simulink model "PioneerROS_Controller"  (R2019b)
settings: Solver=FixedStepAuto  StartTime=0.0  StopTime=inf  FixedStep=0.1  RelTol=1e-3
libraries: robotlib x4
settings Model: SimulationMode=external  EnablePacing=on  Creator=gavin  LastModifiedBy=gavin
settings OptimizationCC: EnhancedBackFolding=on  PassReuseOutputArgsThreshold=0  MaxStackSize=64  OptimizeBlockOrder=speed  DifferentSizesBufferReuse=on  OptimizationCustomize=off
settings DebuggingCC: ParameterTunabilityLossMsg=error
settings HardwareCC: ProdBitPerPointer=32  ProdBitPerSizeT=32  ProdBitPerPtrDiffT=32  ProdLargestAtomicFloat=None  ProdIntDivRoundTo=Undefined  ProdEndianess=Unspecified  ProdWordSize=32  ProdHWDeviceType=Generic->Unspecified (assume 32-bit Generic)  UseEmbeddedCoderFeatures=off
settings SFSimCC: MATLABDynamicMemAlloc=off
settings RTWCC: SystemTargetFile=ert.tlc  HardwareBoard=Robot Operating System (ROS)  TLCOptions="-aInlineSetEventsForThisBaseRateFcn=TLC_FALSE -aSuppressMultiTaskScheduler=TLC_FALSE  -aRateBasedStepFcn=0"  TemplateMakefile=ert_default_tmf  GenerateReport=on  Toolchain=Catkin  LaunchReport=on  TargetLang=C++
settings CodeAppCC: ForceParamTrailComments=on  OperatorAnnotations=on
settings ERTTargetCC: ERTCustomFileBanners=off  SupportContinuousTime=on  SupportNonInlinedSFcns=on  RemoveResetFunc=off  ModelStepFunctionPrototypeControlCompliant=off

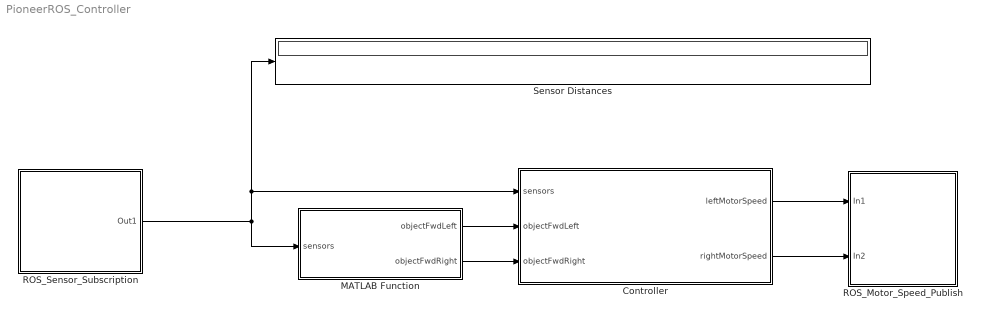
== system PioneerROS_Controller ==
  Controller : Stateflow chart  BlockKeywords=__PRM__SERIALIZED__DATA__:Stateflow Chart,Stateflow Diagram  TreatAsAtomicUnit=on
  MATLAB Function : MATLAB Function  TreatAsAtomicUnit=on
  ROS_Motor_Speed_Publish : Subsystem
  ROS_Sensor_Subscription : Subsystem
  Sensor Distances : Display
  wires:
  ROS_Sensor_Subscription/1(Out1) -> Controller/1(sensors), Sensor Distances/1, MATLAB Function/1(sensors)
  MATLAB Function/1(objectFwdLeft) -> Controller/2(objectFwdLeft)
  MATLAB Function/2(objectFwdRight) -> Controller/3(objectFwdRight)
  Controller/1(leftMotorSpeed) -> ROS_Motor_Speed_Publish/1(In1)
  Controller/2(rightMotorSpeed) -> ROS_Motor_Speed_Publish/2(In2)

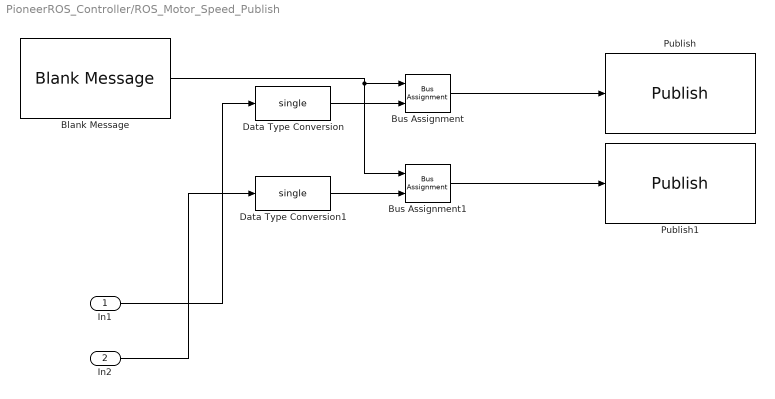
== system PioneerROS_Controller/ROS_Motor_Speed_Publish ==
  In1 : Inport
  In2 : Inport  Port=2
  Blank Message : robotlib/Blank Message  messageClass=Message  entityType=std_msgs/Float32  messageType=std_msgs/Float32  SampleTime=inf
      settings: SourceProductName=ROS Toolbox
  Bus Assignment : BusAssignment  AssignedSignals=Data
  Bus Assignment1 : BusAssignment  AssignedSignals=Data
  Data Type Conversion : DataTypeConversion  OutDataTypeStr=single
  Data Type Conversion1 : DataTypeConversion  OutDataTypeStr=single
  Publish : robotlib/Publish  topicSource=Select from ROS network  topic=/leftMotorSpeed_Bob  messageType=std_msgs/Float32  messageQueueLength=1
      settings: SourceProductName=ROS Toolbox
  Publish1 : robotlib/Publish  topicSource=Select from ROS network  topic=/rightMotorSpeed_Bob  messageType=std_msgs/Float32  messageQueueLength=1
      settings: SourceProductName=ROS Toolbox
  wires:
  In1/1 -> Data Type Conversion/1
  Bus Assignment/1 -> Publish/1
  Data Type Conversion1/1 -> Bus Assignment1/2
  Bus Assignment1/1 -> Publish1/1
  Blank Message/1 -> Bus Assignment1/1, Bus Assignment/1
  Data Type Conversion/1 -> Bus Assignment/2
  In2/1 -> Data Type Conversion1/1

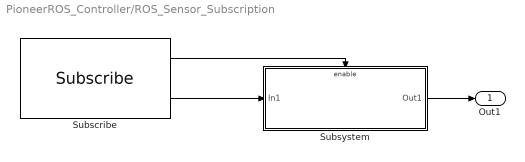
== system PioneerROS_Controller/ROS_Sensor_Subscription ==
  Subscribe : robotlib/Subscribe  topicSource=Select from ROS network  topic=/sensorTrigger_Bob  messageType=std_msgs/Float32MultiArray  sampleTime=0.1  messageQueueLength=1
      settings: SourceProductName=ROS Toolbox
  Subsystem : Subsystem
  Out1 : Outport
  wires:
  Subscribe/2 -> Subsystem/1(In1)
  Subscribe/1 -> Subsystem/Enable
  Subsystem/1(Out1) -> Out1/1

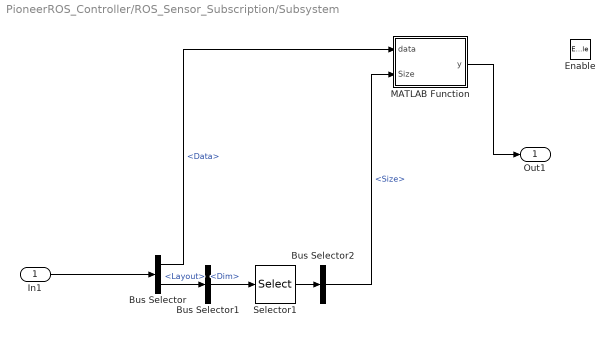
== system PioneerROS_Controller/ROS_Sensor_Subscription/Subsystem ==
  In1 : Inport
  Enable : EnablePort  PropagateVarSize=During execution
  Bus Selector : BusSelector  OutputSignals=Data,Layout
  Bus Selector1 : BusSelector  OutputSignals=Dim
  Bus Selector2 : BusSelector  OutputSignals=Size
  MATLAB Function : MATLAB Function  TreatAsAtomicUnit=on
  Selector1 : Selector  InputPortWidth=16  IndexOptions=Index vector (dialog)  Indices=[1]  OutputSizes=1
  Out1 : Outport
  wires:
  In1/1 -> Bus Selector/1
  Bus Selector1/1 -> Selector1/1  "<Dim>"
  MATLAB Function/1(y) -> Out1/1
  Bus Selector/2 -> Bus Selector1/1  "<Layout>"
  Bus Selector/1 -> MATLAB Function/1(data)  "<Data>"
  Bus Selector2/1 -> MATLAB Function/2(Size)  "<Size>"
  Selector1/1 -> Bus Selector2/1

== matlab function PioneerROS_Controller/MATLAB Function ==
  data: sensors input size=128; objectFwdLeft output size=1; objectFwdRight output size=1
function [objectFwdLeft,objectFwdRight] = fcn(sensors)
if (sensors(1) < 1) || (sensors(2) < 1) || (sensors(3) < 1) || (sensors(4) < 1)
    objectFwdLeft = 1;
else
    objectFwdLeft = 0;
end
if (sensors(5) < 1) || (sensors(6) < 1) || (sensors(7) < 1) || (sensors(8) < 1)
    objectFwdRight = 1;
else
    objectFwdRight = 0;
end

== matlab function PioneerROS_Controller/ROS_Sensor_Subscription/Subsystem/MATLAB Function ==
  data: data input; y output size=128; Size input
function y = fcn(data, Size)
%y = zeros(1,Size);
y = data(1:Size);

== stateflow chart PioneerROS_Controller/Controller ==
  state GoForwards
    en: leftMotorSpeed=1;
    en: rightMotorSpeed=1;
  state GoRight
    en: leftMotorSpeed=0.5;
    en: rightMotorSpeed=-0.5;
  state GoLeft
    en: leftMotorSpeed=-0.5;
    en: rightMotorSpeed=0.5;
  GoLeft -> GoForwards [order 3]
  (default) -> GoForwards
  GoRight -> GoForwards [order 3]
  GoForwards -> GoRight [order 2] : [objectFwdLeft]
  GoForwards -> GoLeft [order 1] : [objectFwdRight]
  GoLeft -> GoRight [order 1] : [objectFwdLeft]
  GoRight -> GoLeft [order 1] : [objectFwdRight]
  GoLeft -> GoLeft [order 2] : [objectFwdRight]
  GoRight -> GoRight [order 2] : [objectFwdLeft]
  data: sensors input size=128; objectFwdLeft input; leftMotorSpeed output single; rightMotorSpeed output single; objectFwdRight input =false
